simulink model "water_4hopper_VDF"  (Simulink 8.0)
settings: Solver=ode23t  StartTime=0.0  StopTime=5  MaxStep=1e-2  RelTol=1e-6
values from neighbouring files (symbols this model uses):
  alpha = 30    [SimParam_4VDF.m]
  amp = leg_length    (= 0.0249)    [SimParam_4VDF.m]
  C_d = 0.703    [SimParam_4VDF.m]
  density = 1000    [SimParam_4VDF.m]
  frame_inertia = diag([Ix,Iy,Iz])    [SimParam_4VDF.m]
  freq = 60    [SimParam_4VDF.m]
  g = 9.81    [SimParam_4VDF.m]
  K_d = 0    [SimParam_4VDF.m]
  K_i = 0    [SimParam_4VDF.m]
  K_p = -50    [SimParam_4VDF.m]
  leg_length = 0.0249    [SimParam_4VDF.m]
  m_toe = 0.0    (= 0)    [SimParam_4VDF.m]
  mass = 0.1    [SimParam_4VDF.m]
  S1 = pi*r1^2*0.9185    (= 0.00115422114093)    [SimParam_4VDF.m]
  S2 = pi*r2^2*0.9185    (= 7.21388213081e-05)    [SimParam_4VDF.m]
  tau = 0.001    [SimParam_4VDF.m]
undefined symbols (not defined in the file): y_0
libraries: mblibv1 x48, powerlib_extras x4, simulink x2
(part 2 of 2)

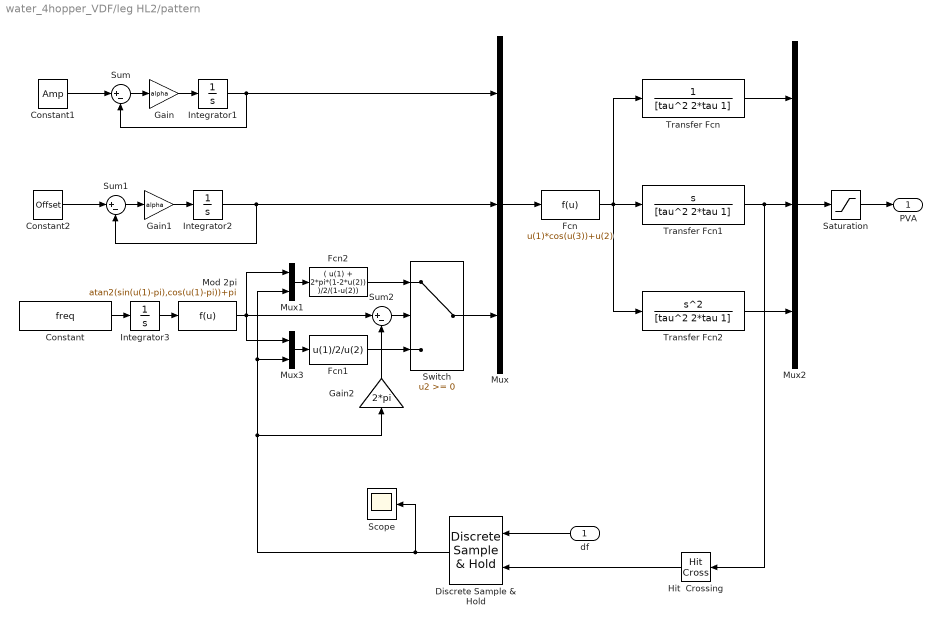
== system water_4hopper_VDF/leg HL2/pattern ==
  df : Inport
  Constant : Constant  Value=freq
  Constant1 : Constant  Value=Amp
  Constant2 : Constant  Value=Offset
  Discrete Sample & Hold : powerlib_extras/Discrete  Control Blocks/Discrete Sample & Hold  ic=0.5  Ts=2/pi/freq/20
  Fcn : Fcn  Expr=u(1)*cos(u(3))+u(2)
  Fcn1 : Fcn  Expr=u(1)/2/u(2)
  Fcn2 : Fcn  Expr=( u(1) + 2*pi*(1-2*u(2)) )/2/(1-u(2))
  Gain : Gain  Gain=alpha
  Gain1 : Gain  Gain=alpha
  Gain2 : Gain  Gain=2*pi
  Hit  Crossing : HitCross  HitCrossingDirection=falling
  Integrator1 : Integrator
  Integrator2 : Integrator
  Integrator3 : Integrator  InitialCondition=0.001*rand
  Mod 2pi : Fcn  Expr=atan2(sin(u(1)-pi),cos(u(1)-pi))+pi
  Mux : Mux  Inputs=3
  Mux1 : Mux  Inputs=2
  Mux2 : Mux  Inputs=3
  Mux3 : Mux  Inputs=2
  Saturation : Saturate  UpperLimit=3*amp*freq^2  LowerLimit=-3*amp*freq^2
  Scope : Scope
  Sum : Sum  Inputs=|+-
  Sum1 : Sum  Inputs=|+-
  Sum2 : Sum  Inputs=|+-
  Switch : Switch
  Transfer Fcn : TransferFcn  Denominator=[tau^2 2*tau 1]
  Transfer Fcn1 : TransferFcn  Numerator=[1 0]  Denominator=[tau^2 2*tau 1]
  Transfer Fcn2 : TransferFcn  Numerator=[1 0 0]  Denominator=[tau^2 2*tau 1]
  PVA : Outport
  wires:
  Constant/1 -> Integrator3/1
  Mod 2pi/1 -> Mux1/1, Mux3/1, Sum2/1
  Integrator3/1 -> Mod 2pi/1
  Switch/1 -> Mux/3
  Fcn1/1 -> Switch/3
  Fcn2/1 -> Switch/1
  Mux/1 -> Fcn/1
  Gain1/1 -> Integrator2/1
  Constant2/1 -> Sum1/1
  Integrator2/1 -> Mux/2, Sum1/2
  Sum1/1 -> Gain1/1
  Gain/1 -> Integrator1/1
  Constant1/1 -> Sum/1
  Integrator1/1 -> Mux/1, Sum/2
  Sum/1 -> Gain/1
  Transfer Fcn2/1 -> Mux2/3
  Transfer Fcn/1 -> Mux2/1
  Transfer Fcn1/1 -> Hit  Crossing/1, Mux2/2
  Mux2/1 -> Saturation/1
  Fcn/1 -> Transfer Fcn1/1, Transfer Fcn/1, Transfer Fcn2/1
  Saturation/1 -> PVA/1
  Hit  Crossing/1 -> Discrete Sample & Hold/2
  Sum2/1 -> Switch/2
  Gain2/1 -> Sum2/2
  Discrete Sample & Hold/1 -> Scope/1, Mux3/2, Mux1/2, Gain2/1
  Mux1/1 -> Fcn2/1
  Mux3/1 -> Fcn1/1
  df/1 -> Discrete Sample & Hold/1

== system water_4hopper_VDF/leg HL3/Subsystem ==
  pos : Inport
  vel : Inport  Port=2
  Constant : Constant  Value=0
  Gain : Gain  Gain=C_d*density
  Gain1 : Gain  Gain=-0.5
  Gain2 : Gain  Gain=S1
  Gain3 : Gain  Gain=g
  Gain4 : Gain  Gain=S2
  Gain5 : Gain  Gain=0.5
  Math Function : Math  Operator=square  SaturateOnIntegerOverflow=on
  Sum : Sum  Inputs=-+|
  Sum1 : Sum  Inputs=-+|
  Switch : Switch  ZeroCross=off
  Switch1 : Switch
  force : Outport
  wires:
  Gain5/1 -> Sum1/2
  Sum1/1 -> Gain2/1
  Constant/1 -> Switch1/1
  Gain/1 -> Switch1/3
  Switch1/1 -> force/1
  Switch/1 -> Gain/1
  Gain2/1 -> Switch/3
  Gain4/1 -> Switch/1
  Sum/1 -> Gain4/1
  Gain3/1 -> Sum1/1, Sum/1
  pos/1 -> Switch1/2, Gain3/1
  Gain1/1 -> Sum/2
  Math Function/1 -> Gain5/1, Gain1/1
  vel/1 -> Math Function/1, Switch/2

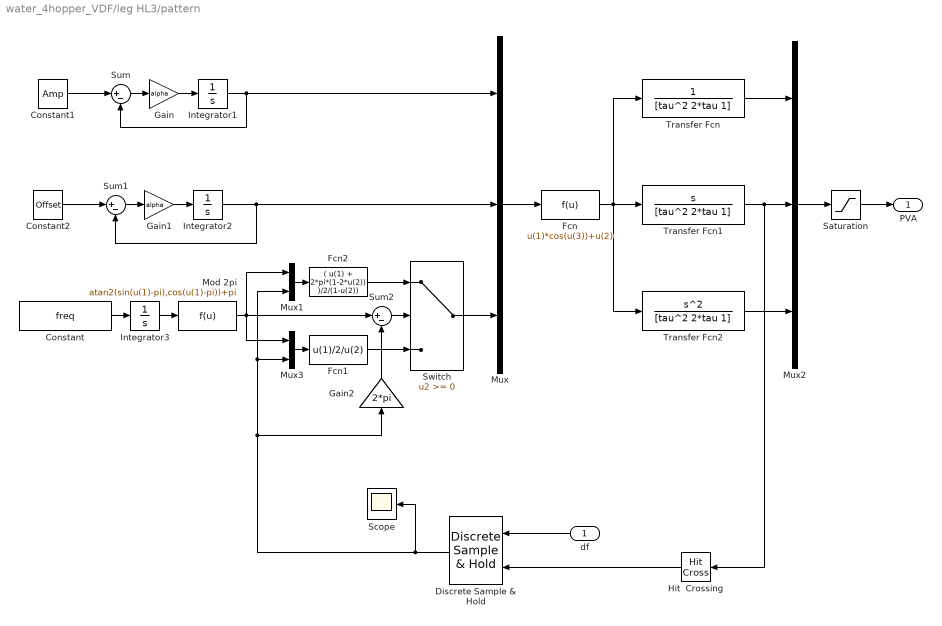
== system water_4hopper_VDF/leg HL3/pattern ==
  df : Inport
  Constant : Constant  Value=freq
  Constant1 : Constant  Value=Amp
  Constant2 : Constant  Value=Offset
  Discrete Sample & Hold : powerlib_extras/Discrete  Control Blocks/Discrete Sample & Hold  ic=0.5  Ts=2/pi/freq/20
  Fcn : Fcn  Expr=u(1)*cos(u(3))+u(2)
  Fcn1 : Fcn  Expr=u(1)/2/u(2)
  Fcn2 : Fcn  Expr=( u(1) + 2*pi*(1-2*u(2)) )/2/(1-u(2))
  Gain : Gain  Gain=alpha
  Gain1 : Gain  Gain=alpha
  Gain2 : Gain  Gain=2*pi
  Hit  Crossing : HitCross  HitCrossingDirection=falling
  Integrator1 : Integrator
  Integrator2 : Integrator
  Integrator3 : Integrator  InitialCondition=0.001*rand
  Mod 2pi : Fcn  Expr=atan2(sin(u(1)-pi),cos(u(1)-pi))+pi
  Mux : Mux  Inputs=3
  Mux1 : Mux  Inputs=2
  Mux2 : Mux  Inputs=3
  Mux3 : Mux  Inputs=2
  Saturation : Saturate  UpperLimit=3*amp*freq^2  LowerLimit=-3*amp*freq^2
  Scope : Scope
  Sum : Sum  Inputs=|+-
  Sum1 : Sum  Inputs=|+-
  Sum2 : Sum  Inputs=|+-
  Switch : Switch
  Transfer Fcn : TransferFcn  Denominator=[tau^2 2*tau 1]
  Transfer Fcn1 : TransferFcn  Numerator=[1 0]  Denominator=[tau^2 2*tau 1]
  Transfer Fcn2 : TransferFcn  Numerator=[1 0 0]  Denominator=[tau^2 2*tau 1]
  PVA : Outport
  wires:
  Constant/1 -> Integrator3/1
  Mod 2pi/1 -> Mux1/1, Mux3/1, Sum2/1
  Integrator3/1 -> Mod 2pi/1
  Switch/1 -> Mux/3
  Fcn1/1 -> Switch/3
  Fcn2/1 -> Switch/1
  Mux/1 -> Fcn/1
  Gain1/1 -> Integrator2/1
  Constant2/1 -> Sum1/1
  Integrator2/1 -> Mux/2, Sum1/2
  Sum1/1 -> Gain1/1
  Gain/1 -> Integrator1/1
  Constant1/1 -> Sum/1
  Integrator1/1 -> Mux/1, Sum/2
  Sum/1 -> Gain/1
  Transfer Fcn2/1 -> Mux2/3
  Transfer Fcn/1 -> Mux2/1
  Transfer Fcn1/1 -> Hit  Crossing/1, Mux2/2
  Mux2/1 -> Saturation/1
  Fcn/1 -> Transfer Fcn1/1, Transfer Fcn/1, Transfer Fcn2/1
  Saturation/1 -> PVA/1
  Hit  Crossing/1 -> Discrete Sample & Hold/2
  Sum2/1 -> Switch/2
  Gain2/1 -> Sum2/2
  Discrete Sample & Hold/1 -> Scope/1, Mux3/2, Mux1/2, Gain2/1
  Mux1/1 -> Fcn2/1
  Mux3/1 -> Fcn1/1
  df/1 -> Discrete Sample & Hold/1
